simulink model "audio_setup"  (R2019b)
settings: Solver=FixedStepDiscrete  StartTime=0.0  StopTime=0.1  RelTol=1e-3
undefined symbols (not defined in the file): DiscIntNeverNeededParam
libraries: hdlsllib x15, simulink x11
settings Model: DataTypeOverride=Off  Creator=shahryar  LastModifiedBy=shahryar
settings SolverCC: AutoInsertRateTranBlk=on
settings DataIOCC: LimitDataPoints=on  SaveOutput=off  SaveTime=off
settings OptimizationCC: BlockReduction=off  ConditionallyExecuteInputs=off  DefaultParameterBehavior=Inlined  LifeSpan=inf
settings DebuggingCC: SignalRangeChecking=warning  AlgebraicLoopMsg=error  SingleTaskRateTransMsg=error  AllowSymbolicDim=off  StrictBusMsg=ErrorOnBusTreatedAsVector  SFUnexpectedBacktrackingDiag=warning  SFNoUnconditionalDefaultTransitionDiag=warning  SFExecutionAtInitializationDiag=none  ArithmeticOperatorsInVariantConditions=warning
settings HardwareCC: ProdBitPerPointer=32  ProdBitPerSizeT=32  ProdBitPerPtrDiffT=32  ProdLargestAtomicFloat=None  ProdIntDivRoundTo=Undefined  ProdEndianess=Unspecified  ProdWordSize=32  ProdHWDeviceType=ASIC/FPGA->ASIC/FPGA  TargetBitPerLong=64  TargetBitPerPointer=64  TargetBitPerSizeT=64  TargetBitPerPtrDiffT=64  TargetLongLongMode=on  TargetIntDivRoundTo=Zero  TargetEndianess=LittleEndian  TargetWordSize=64  TargetHWDeviceType=Custom Processor->MATLAB Host Computer  ProdEqTarget=off
settings SFSimCC: SimUseLocalCustomCode=off  CustomCodeUndefinedFunction=UseInterfaceOnly
settings RTWCC: RTWUseLocalCustomCode=off
settings CodeAppCC: StateflowObjectComments=on
settings GRTTargetCC: TargetLangStandard=C89/C90 (ANSI)  GeneratePreprocessorConditionals=Disable all
settings ConfigComp: CovScope=ReferencedModels  CovMetricSettings=dw  CovHtmlReporting=on  CovSaveCumulativeToWorkspaceVar=on  CovSaveSingleToWorkspaceVar=on  CovExternalEMLEnable=off  CovSFcnEnable=off

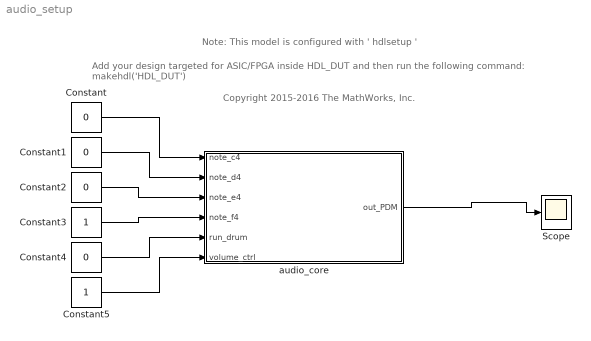
== system audio_setup ==
  note: Note: This model is configured with ' hdlsetup '
  note: Add your design targeted for ASIC/FPGA inside HDL_DUT and then run the following command:
      | makehdl('HDL_DUT')
  note: Copyright 2015-2016 The MathWorks, Inc.
  Constant{,1..2,4} (4 alike) : Constant  Value=0  OutDataTypeStr=boolean  SampleTime=1e-08
  Constant3 : Constant  OutDataTypeStr=boolean  SampleTime=1e-08
  Constant5 : Constant  OutDataTypeStr=fixdt(0,8,8)  SampleTime=1e-08
  Scope : Scope
  audio_core : Subsystem
  wires:
  Constant/1 -> audio_core/1(note_c4)
  Constant1/1 -> audio_core/2(note_d4)
  Constant2/1 -> audio_core/3(note_e4)
  Constant3/1 -> audio_core/4(note_f4)
  Constant4/1 -> audio_core/5(run_drum)
  Constant5/1 -> audio_core/6(volume_ctrl)
  audio_core/1(out_PDM) -> Scope/1

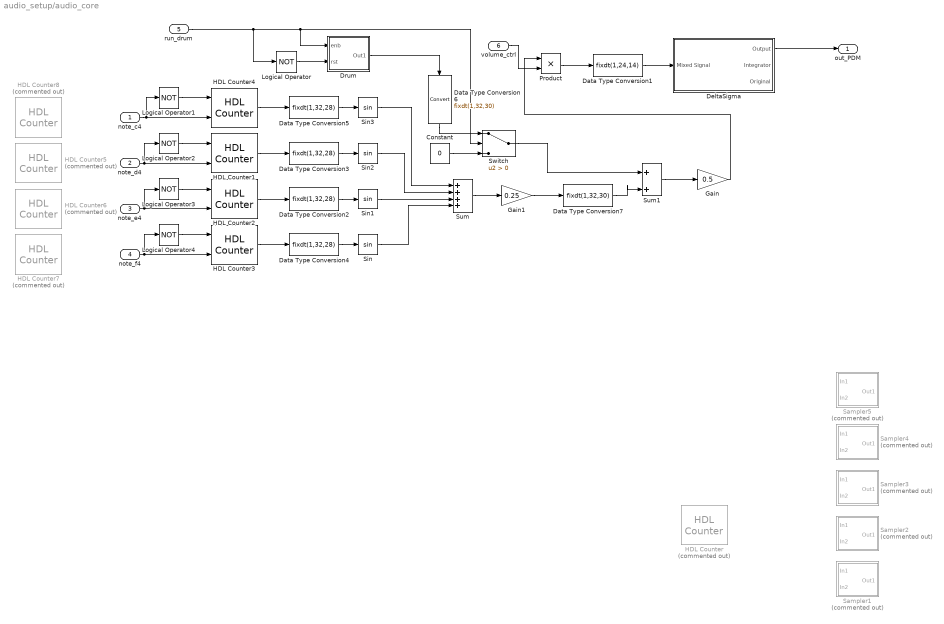
== system audio_setup/audio_core ==
  note_c4 : Inport
  note_d4 : Inport  Port=2
  note_e4 : Inport  Port=3
  note_f4 : Inport  Port=4
  run_drum : Inport  Port=5
  volume_ctrl : Inport  Port=6  OutDataTypeStr=fixdt(0,8,8)
  Constant : Constant  Value=0  OutDataTypeStr=fixdt(1,32,30)  SampleTime=1e-08
  Data Type Conversion1 : DataTypeConversion  OutDataTypeStr=fixdt(1,24,14)
  Data Type Conversion{2..5} (4 alike) : DataTypeConversion  OutDataTypeStr=fixdt(1,32,28)  ConvertRealWorld=Stored Integer (SI)
  Data Type Conversion6 : DataTypeConversion  OutDataTypeStr=fixdt(1,32,30)
  Data Type Conversion7 : DataTypeConversion  OutDataTypeStr=fixdt(1,32,30)
  DeltaSigma : Subsystem
  Drum : Subsystem
  Gain : Gain  Gain=0.5
  Gain1 : Gain  Gain=0.25
  HDL Counter : hdlsllib/Sources/HDL Counter  Commented=on  CountType=Count limited  CountInit=0  CountStep=1  CountMax=9  CountFromType=Initial value  CountFrom=0  CountResetPort=off  CountLoadPort=off  CountEnbPort=off  CountDirPort=off  CountDataType=Unsigned  CountWordLen=16  CountFracLen=0  CountSampTime=1e-08
      settings: SourceProductName=Simulink
  HDL Counter1 : hdlsllib/Sources/HDL Counter  CountType=Count limited  CountInit=3451652439+2218  CountStep=4953  CountMax=843314857-2218  CountFromType=Initial value  CountFrom=3451652439+2218  CountResetPort=on  CountLoadPort=off  CountEnbPort=on  CountDirPort=off  CountDataType=Unsigned  CountWordLen=32  CountFracLen=0  CountSampTime=1e-07
      settings: SourceProductName=Simulink
  HDL Counter2 : hdlsllib/Sources/HDL Counter  CountType=Count limited  CountInit=3451652439+1857  CountStep=5560  CountMax=843314857-1857  CountFromType=Initial value  CountFrom=3451652439+1857  CountResetPort=on  CountLoadPort=off  CountEnbPort=on  CountDirPort=off  CountDataType=Unsigned  CountWordLen=32  CountFracLen=0  CountSampTime=1e-07
      settings: SourceProductName=Simulink
  HDL Counter3 : hdlsllib/Sources/HDL Counter  CountType=Count limited  CountInit=3451652439+2327  CountStep=5890  CountMax=843314857-2327  CountFromType=Initial value  CountFrom=3451652439+2327  CountResetPort=on  CountLoadPort=off  CountEnbPort=on  CountDirPort=off  CountDataType=Unsigned  CountWordLen=32  CountFracLen=0  CountSampTime=1e-07
      settings: SourceProductName=Simulink
  HDL Counter4 : hdlsllib/Sources/HDL Counter  CountType=Count limited  CountInit=3451652439+1590  CountStep=4413  CountMax=843314857-1589  CountFromType=Initial value  CountFrom=3451652439+1590  CountResetPort=on  CountLoadPort=off  CountEnbPort=on  CountDirPort=off  CountDataType=Unsigned  CountWordLen=32  CountFracLen=0  CountSampTime=1e-07
      settings: SourceProductName=Simulink
  HDL Counter5 : hdlsllib/Sources/HDL Counter  Commented=on  CountType=Count limited  CountInit=3451652439+7171  CountStep=19812  CountMax=843314857-7171  CountFromType=Initial value  CountFrom=3451652439+7171  CountResetPort=on  CountLoadPort=off  CountEnbPort=on  CountDirPort=off  CountDataType=Unsigned  CountWordLen=32  CountFracLen=0  CountSampTime=1e-07
      settings: SourceProductName=Simulink
  HDL Counter6 : hdlsllib/Sources/HDL Counter  Commented=on  CountType=Count limited  CountInit=3451652439+5421  CountStep=22238  CountMax=843314857-5421  CountFromType=Initial value  CountFrom=3451652439+5421  CountResetPort=on  CountLoadPort=off  CountEnbPort=on  CountDirPort=off  CountDataType=Unsigned  CountWordLen=32  CountFracLen=0  CountSampTime=1e-07
      settings: SourceProductName=Simulink
  HDL Counter7 : hdlsllib/Sources/HDL Counter  Commented=on  CountType=Count limited  CountInit=3451652439+7765  CountStep=23561  CountMax=843314857-7764  CountFromType=Initial value  CountFrom=3451652439+7765  CountResetPort=on  CountLoadPort=off  CountEnbPort=on  CountDirPort=off  CountDataType=Unsigned  CountWordLen=32  CountFracLen=0  CountSampTime=1e-07
      settings: SourceProductName=Simulink
  HDL Counter8 : hdlsllib/Sources/HDL Counter  Commented=on  CountType=Count limited  CountInit=3451652439+3030  CountStep=17651  CountMax=843314857-3030  CountFromType=Initial value  CountFrom=3451652439+3030  CountResetPort=on  CountLoadPort=off  CountEnbPort=on  CountDirPort=off  CountDataType=Unsigned  CountWordLen=32  CountFracLen=0  CountSampTime=1e-07
      settings: SourceProductName=Simulink
  Logical Operator{,1..4} (5 alike) : Logic  Operator=NOT  IconShape=distinctive  AllPortsSameDT=off  OutDataTypeStr=boolean
  Product : Product
  Sampler1 : Subsystem  Commented=on
  Sampler2 : Subsystem  Commented=on
  Sampler3 : Subsystem  Commented=on
  Sampler4 : Subsystem  Commented=on
  Sampler5 : Subsystem  Commented=on
  Sin{,1..3} (4 alike) : Trigonometry  ApproximationMethod=CORDIC  NumberOfIterations=5  OutputSignalType=real
  Sum : Sum  Inputs=|+|+|+|+|
  Sum1 : Sum  Inputs=|+|+|
  Switch : Switch  Criteria=u2 > Threshold
  out_PDM : Outport  VectorParamsAs1DForOutWhenUnconnected=off
  wires:
  Data Type Conversion1/1 -> DeltaSigma/1(Mixed Signal)
  note_f4/1 -> Logical Operator4/1, HDL Counter3/2
  HDL Counter3/1 -> Data Type Conversion4/1
  Data Type Conversion4/1 -> Sin/1
  DeltaSigma/1(Output) -> out_PDM/1
  note_e4/1 -> Logical Operator3/1, HDL Counter2/2
  Data Type Conversion2/1 -> Sin1/1
  note_d4/1 -> Logical Operator2/1, HDL Counter1/2
  Data Type Conversion3/1 -> Sin2/1
  note_c4/1 -> Logical Operator1/1, HDL Counter4/2
  HDL Counter2/1 -> Data Type Conversion2/1
  HDL Counter1/1 -> Data Type Conversion3/1
  HDL Counter4/1 -> Data Type Conversion5/1
  Data Type Conversion5/1 -> Sin3/1
  run_drum/1 -> Logical Operator/1, Drum/1(enb), Switch/2
  Data Type Conversion6/1 -> Switch/1
  Constant/1 -> Switch/3
  Logical Operator1/1 -> HDL Counter4/1
  Logical Operator4/1 -> HDL Counter3/1
  Logical Operator3/1 -> HDL Counter2/1
  Logical Operator2/1 -> HDL Counter1/1
  Drum/1(Out1) -> Data Type Conversion6/1
  Logical Operator/1 -> Drum/2(rst)
  Gain/1 -> Product/1
  volume_ctrl/1 -> Product/2
  Product/1 -> Data Type Conversion1/1
  Sin3/1 -> Sum/1
  Sin2/1 -> Sum/2
  Sin1/1 -> Sum/3
  Sin/1 -> Sum/4
  Sum/1 -> Gain1/1
  Switch/1 -> Sum1/1
  Sum1/1 -> Gain/1
  Gain1/1 -> Data Type Conversion7/1
  Data Type Conversion7/1 -> Sum1/2

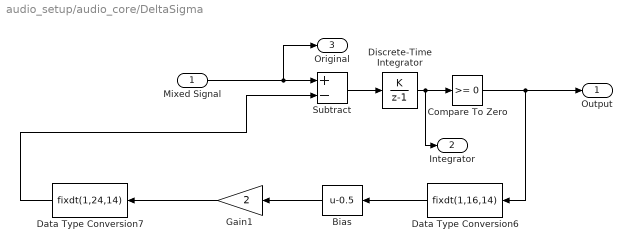
== system audio_setup/audio_core/DeltaSigma ==
  Mixed Signal : Inport
  Bias : Bias  Bias=-0.5
  Compare To Zero : simulink/Logic and Bit Operations/Compare To Zero  relop=>=  OutDataTypeStr=boolean
  Data Type Conversion6 : DataTypeConversion  OutDataTypeStr=fixdt(1,16,14)
  Data Type Conversion7 : DataTypeConversion  OutDataTypeStr=fixdt(1,24,14)
  Discrete-Time Integrator : DiscreteIntegrator  IntegratorMethod=Accumulation: Forward Euler  gainval=1  SampleTime=-1  OutDataTypeStr=fixdt(1,24,14)  UpperSaturationLimit=1  LowerSaturationLimit=-1  ICPrevOutput=DiscIntNeverNeededParam  ICPrevScaledInput=DiscIntNeverNeededParam
  Gain1 : Gain  Gain=2
  Subtract : Sum  Inputs=+-  AccumDataTypeStr=fixdt(1,16,12)  InputSameDT=on
  Output : Outport
  Integrator : Outport  Port=2  VectorParamsAs1DForOutWhenUnconnected=off
  Original : Outport  Port=3  VectorParamsAs1DForOutWhenUnconnected=off
  wires:
  Gain1/1 -> Data Type Conversion7/1
  Bias/1 -> Gain1/1
  Compare To Zero/1 -> Output/1, Data Type Conversion6/1
  Mixed Signal/1 -> Original/1, Subtract/1
  Data Type Conversion6/1 -> Bias/1
  Data Type Conversion7/1 -> Subtract/2
  Subtract/1 -> Discrete-Time Integrator/1
  Discrete-Time Integrator/1 -> Integrator/1, Compare To Zero/1

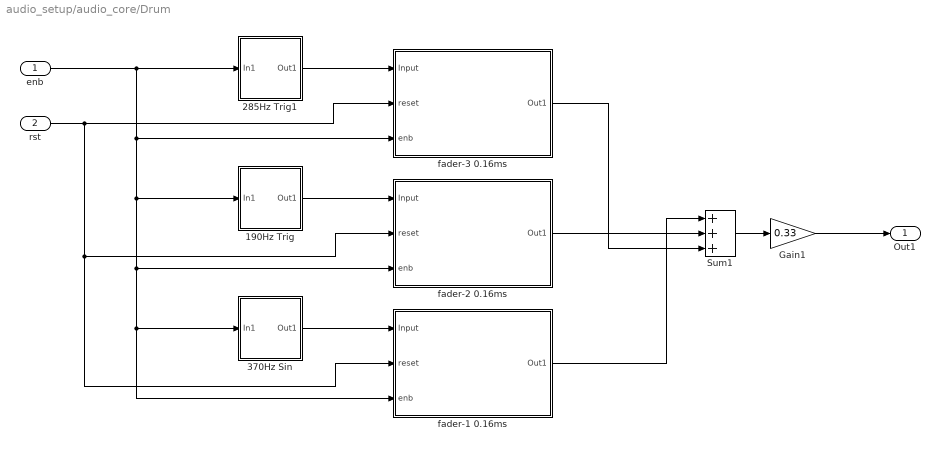
== system audio_setup/audio_core/Drum ==
  enb : Inport
  rst : Inport  Port=2
  190Hz Trig : Subsystem
  285Hz Trig1 : Subsystem
  370Hz Sin : Subsystem
  Gain1 : Gain  Gain=0.33
  Sum1 : Sum  Inputs=|+|+|+|
  fader-1 0.16ms : Subsystem
  fader-2 0.16ms : Subsystem
  fader-3 0.16ms : Subsystem
  Out1 : Outport
  wires:
  285Hz Trig1/1(Out1) -> fader-3 0.16ms/1(Input)
  Sum1/1 -> Gain1/1
  fader-2 0.16ms/1(Out1) -> Sum1/2
  370Hz Sin/1(Out1) -> fader-1 0.16ms/1(Input)
  190Hz Trig/1(Out1) -> fader-2 0.16ms/1(Input)
  fader-1 0.16ms/1(Out1) -> Sum1/1
  Gain1/1 -> Out1/1
  enb/1 -> 190Hz Trig/1(In1), fader-2 0.16ms/3(enb), fader-1 0.16ms/3(enb), 370Hz Sin/1(In1), fader-3 0.16ms/3(enb), 285Hz Trig1/1(In1)
  rst/1 -> fader-1 0.16ms/2(reset), fader-2 0.16ms/2(reset), fader-3 0.16ms/2(reset)
  fader-3 0.16ms/1(Out1) -> Sum1/3

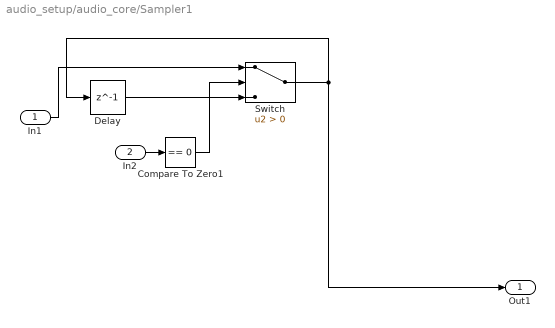
== system audio_setup/audio_core/Sampler1 ==
  In1 : Inport
  In2 : Inport  Port=2
  Compare To Zero1 : simulink/Logic and Bit Operations/Compare To Zero  relop===  OutDataTypeStr=boolean
  Delay : Delay  DelayLength=1  InitialCondition=1  UseCircularBuffer=on
  Switch : Switch  Criteria=u2 > Threshold
  Out1 : Outport
  wires:
  Delay/1 -> Switch/3
  In2/1 -> Compare To Zero1/1
  In1/1 -> Switch/1
  Switch/1 -> Out1/1, Delay/1
  Compare To Zero1/1 -> Switch/2

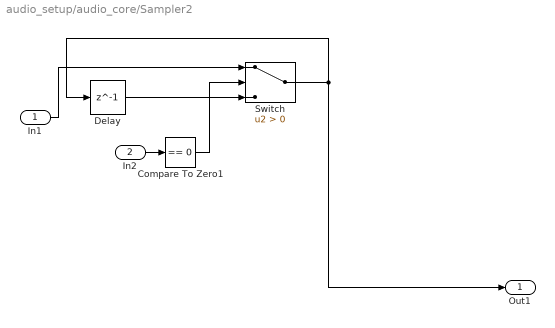
== system audio_setup/audio_core/Sampler2 ==
  In1 : Inport
  In2 : Inport  Port=2
  Compare To Zero1 : simulink/Logic and Bit Operations/Compare To Zero  relop===  OutDataTypeStr=boolean
  Delay : Delay  DelayLength=1  InitialCondition=1  UseCircularBuffer=on
  Switch : Switch  Criteria=u2 > Threshold
  Out1 : Outport
  wires:
  Delay/1 -> Switch/3
  In2/1 -> Compare To Zero1/1
  In1/1 -> Switch/1
  Switch/1 -> Out1/1, Delay/1
  Compare To Zero1/1 -> Switch/2

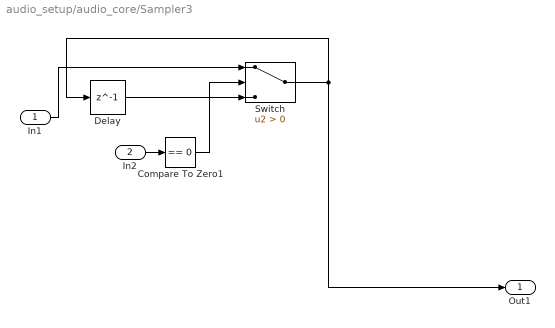
== system audio_setup/audio_core/Sampler3 ==
  In1 : Inport
  In2 : Inport  Port=2
  Compare To Zero1 : simulink/Logic and Bit Operations/Compare To Zero  relop===  OutDataTypeStr=boolean
  Delay : Delay  DelayLength=1  InitialCondition=1  UseCircularBuffer=on
  Switch : Switch  Criteria=u2 > Threshold
  Out1 : Outport
  wires:
  Delay/1 -> Switch/3
  In2/1 -> Compare To Zero1/1
  In1/1 -> Switch/1
  Switch/1 -> Out1/1, Delay/1
  Compare To Zero1/1 -> Switch/2

== system audio_setup/audio_core/Sampler4 ==
  In1 : Inport
  In2 : Inport  Port=2
  Compare To Zero1 : simulink/Logic and Bit Operations/Compare To Zero  relop===  OutDataTypeStr=boolean
  Delay : Delay  DelayLength=1  InitialCondition=1  UseCircularBuffer=on
  Switch : Switch  Criteria=u2 > Threshold
  Out1 : Outport
  wires:
  Delay/1 -> Switch/3
  In2/1 -> Compare To Zero1/1
  In1/1 -> Switch/1
  Switch/1 -> Out1/1, Delay/1
  Compare To Zero1/1 -> Switch/2

== system audio_setup/audio_core/Sampler5 ==
  In1 : Inport
  In2 : Inport  Port=2
  Compare To Zero1 : simulink/Logic and Bit Operations/Compare To Zero  relop===  OutDataTypeStr=boolean
  Delay : Delay  DelayLength=1  InitialCondition=1  UseCircularBuffer=on
  Switch : Switch  Criteria=u2 > Threshold
  Out1 : Outport
  wires:
  Delay/1 -> Switch/3
  In2/1 -> Compare To Zero1/1
  In1/1 -> Switch/1
  Switch/1 -> Out1/1, Delay/1
  Compare To Zero1/1 -> Switch/2

== system audio_setup/audio_core/Drum/190Hz Trig ==
  In1 : Inport
  Data Type Conversion6 : DataTypeConversion  OutDataTypeStr=fixdt(1,22,18)  ConvertRealWorld=Stored Integer (SI)
  Data Type Conversion7 : DataTypeConversion  OutDataTypeStr=fixdt(1,20,16)
  HDL Counter6 : hdlsllib/Sources/HDL Counter  CountType=Count limited  CountInit=0  CountStep=1  CountMax=262144  CountFromType=Initial value  CountFrom=0  CountResetPort=off  CountLoadPort=off  CountEnbPort=on  CountDirPort=off  CountDataType=Unsigned  CountWordLen=22  CountFracLen=0  CountSampTime=1
      settings: SourceProductName=Simulink
  Trig1 : Subsystem
  Out1 : Outport
  wires:
  In1/1 -> HDL Counter6/1
  HDL Counter6/1 -> Trig1/1(In1), Data Type Conversion6/1
  Data Type Conversion6/1 -> Trig1/2(In2)
  Data Type Conversion7/1 -> Out1/1
  Trig1/1(Out1) -> Data Type Conversion7/1

== system audio_setup/audio_core/Drum/285Hz Trig1 ==
  In1 : Inport
  Data Type Conversion6 : DataTypeConversion  OutDataTypeStr=fixdt(1,23,19)  ConvertRealWorld=Stored Integer (SI)
  Data Type Conversion7 : DataTypeConversion  OutDataTypeStr=fixdt(1,20,16)
  HDL Counter6 : hdlsllib/Sources/HDL Counter  CountType=Count limited  CountInit=0  CountStep=3  CountMax=524286  CountFromType=Initial value  CountFrom=0  CountResetPort=off  CountLoadPort=off  CountEnbPort=on  CountDirPort=off  CountDataType=Unsigned  CountWordLen=23  CountFracLen=0  CountSampTime=1
      settings: SourceProductName=Simulink
  Trig1 : Subsystem
  Out1 : Outport
  wires:
  In1/1 -> HDL Counter6/1
  HDL Counter6/1 -> Trig1/1(In1), Data Type Conversion6/1
  Data Type Conversion6/1 -> Trig1/2(In2)
  Data Type Conversion7/1 -> Out1/1
  Trig1/1(Out1) -> Data Type Conversion7/1

== system audio_setup/audio_core/Drum/370Hz Sin ==
  In1 : Inport
  Data Type Conversion6 : DataTypeConversion  OutDataTypeStr=fixdt(1,21,17)  ConvertRealWorld=Stored Integer (SI)
  Data Type Conversion7 : DataTypeConversion  OutDataTypeStr=fixdt(1,20,18)
  HDL Counter5 : hdlsllib/Sources/HDL Counter  CountType=Count limited  CountInit=1685377  CountStep=3  CountMax=411773  CountFromType=Initial value  CountFrom=1685377  CountResetPort=off  CountLoadPort=off  CountEnbPort=on  CountDirPort=off  CountDataType=Unsigned  CountWordLen=21  CountFracLen=0  CountSampTime=1e-07
      settings: SourceProductName=Simulink
  Sin4 : Trigonometry  ApproximationMethod=CORDIC  NumberOfIterations=5  OutputSignalType=real
  Out1 : Outport
  wires:
  HDL Counter5/1 -> Data Type Conversion6/1
  Sin4/1 -> Data Type Conversion7/1
  Data Type Conversion6/1 -> Sin4/1
  In1/1 -> HDL Counter5/1
  Data Type Conversion7/1 -> Out1/1

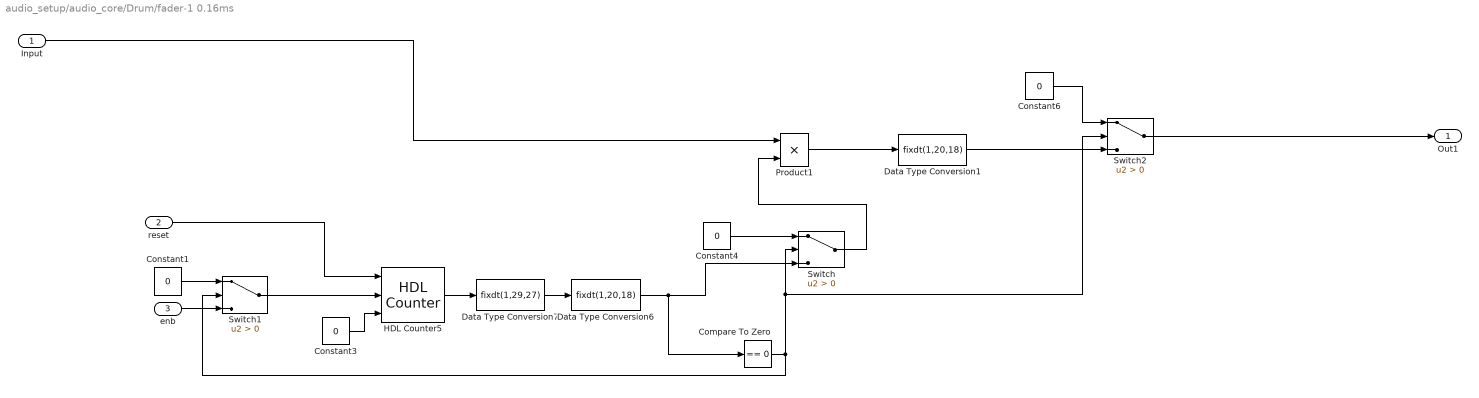
== system audio_setup/audio_core/Drum/fader-1 0.16ms ==
  Input : Inport
  reset : Inport  Port=2
  enb : Inport  Port=3
  Compare To Zero : simulink/Logic and Bit Operations/Compare To Zero  relop===  OutDataTypeStr=boolean
  Constant1 : Constant  Value=0  OutDataTypeStr=boolean  SampleTime=1e-08
  Constant3 : Constant  Value=0  OutDataTypeStr=boolean  SampleTime=1e-08
  Constant4 : Constant  Value=0  OutDataTypeStr=fixdt(1,20,18)  SampleTime=1e-08
  Constant6 : Constant  Value=0  OutDataTypeStr=fixdt(1,20,18)  SampleTime=1e-08
  Data Type Conversion1 : DataTypeConversion  OutDataTypeStr=fixdt(1,20,18)
  Data Type Conversion6 : DataTypeConversion  OutDataTypeStr=fixdt(1,20,18)
  Data Type Conversion7 : DataTypeConversion  OutDataTypeStr=fixdt(1,29,27)  ConvertRealWorld=Stored Integer (SI)
  HDL Counter5 : hdlsllib/Sources/HDL Counter  CountType=Count limited  CountInit=134217728  CountStep=8  CountMax=0  CountFromType=Specify  CountFrom=134217728  CountResetPort=on  CountLoadPort=off  CountEnbPort=on  CountDirPort=on  CountDataType=Unsigned  CountWordLen=29  CountFracLen=0  CountSampTime=1e-07
      settings: SourceProductName=Simulink
  Product1 : Product
  Switch : Switch  Criteria=u2 > Threshold
  Switch1 : Switch  Criteria=u2 > Threshold
  Switch2 : Switch  Criteria=u2 > Threshold
  Out1 : Outport
  wires:
  Switch/1 -> Product1/2
  Data Type Conversion6/1 -> Compare To Zero/1, Switch/3
  Compare To Zero/1 -> Switch2/2, Switch/2, Switch1/2
  Constant6/1 -> Switch2/1
  Data Type Conversion7/1 -> Data Type Conversion6/1
  Constant4/1 -> Switch/1
  Switch1/1 -> HDL Counter5/2
  Switch2/1 -> Out1/1
  Input/1 -> Product1/1
  reset/1 -> HDL Counter5/1
  HDL Counter5/1 -> Data Type Conversion7/1
  Constant3/1 -> HDL Counter5/3
  Constant1/1 -> Switch1/1
  enb/1 -> Switch1/3
  Product1/1 -> Data Type Conversion1/1
  Data Type Conversion1/1 -> Switch2/3

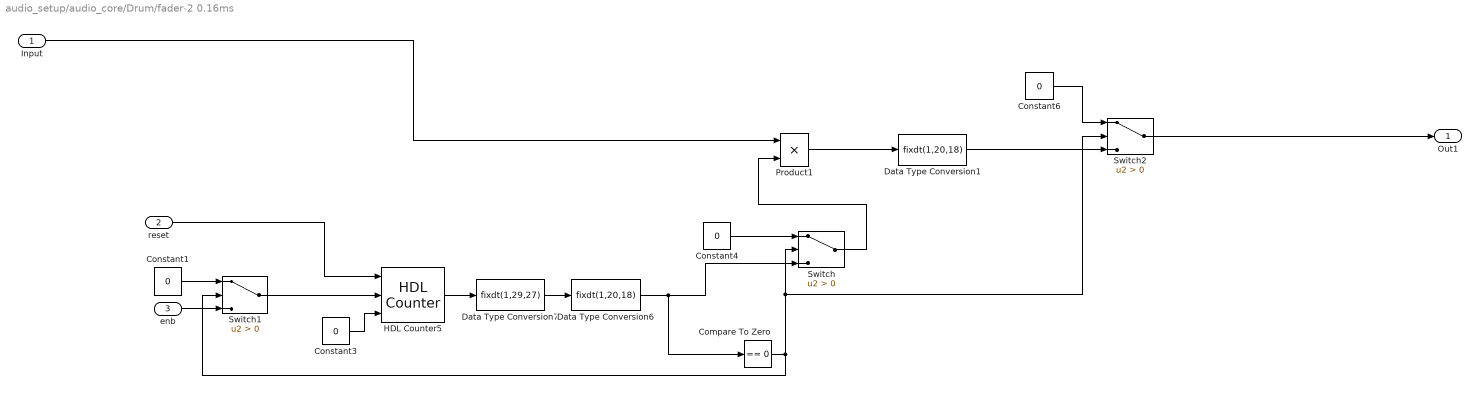
== system audio_setup/audio_core/Drum/fader-2 0.16ms ==
  Input : Inport
  reset : Inport  Port=2
  enb : Inport  Port=3
  Compare To Zero : simulink/Logic and Bit Operations/Compare To Zero  relop===  OutDataTypeStr=boolean
  Constant1 : Constant  Value=0  OutDataTypeStr=boolean  SampleTime=1e-08
  Constant3 : Constant  Value=0  OutDataTypeStr=boolean  SampleTime=1e-08
  Constant4 : Constant  Value=0  OutDataTypeStr=fixdt(1,20,18)  SampleTime=1e-08
  Constant6 : Constant  Value=0  OutDataTypeStr=fixdt(1,20,18)  SampleTime=1e-08
  Data Type Conversion1 : DataTypeConversion  OutDataTypeStr=fixdt(1,20,18)
  Data Type Conversion6 : DataTypeConversion  OutDataTypeStr=fixdt(1,20,18)
  Data Type Conversion7 : DataTypeConversion  OutDataTypeStr=fixdt(1,29,27)  ConvertRealWorld=Stored Integer (SI)
  HDL Counter5 : hdlsllib/Sources/HDL Counter  CountType=Count limited  CountInit=134217728  CountStep=8  CountMax=0  CountFromType=Specify  CountFrom=134217728  CountResetPort=on  CountLoadPort=off  CountEnbPort=on  CountDirPort=on  CountDataType=Unsigned  CountWordLen=29  CountFracLen=0  CountSampTime=1e-07
      settings: SourceProductName=Simulink
  Product1 : Product
  Switch : Switch  Criteria=u2 > Threshold
  Switch1 : Switch  Criteria=u2 > Threshold
  Switch2 : Switch  Criteria=u2 > Threshold
  Out1 : Outport
  wires:
  Switch/1 -> Product1/2
  Data Type Conversion6/1 -> Compare To Zero/1, Switch/3
  Compare To Zero/1 -> Switch2/2, Switch/2, Switch1/2
  Constant6/1 -> Switch2/1
  Data Type Conversion7/1 -> Data Type Conversion6/1
  Constant4/1 -> Switch/1
  Switch1/1 -> HDL Counter5/2
  Switch2/1 -> Out1/1
  Input/1 -> Product1/1
  reset/1 -> HDL Counter5/1
  HDL Counter5/1 -> Data Type Conversion7/1
  Constant3/1 -> HDL Counter5/3
  Constant1/1 -> Switch1/1
  enb/1 -> Switch1/3
  Product1/1 -> Data Type Conversion1/1
  Data Type Conversion1/1 -> Switch2/3

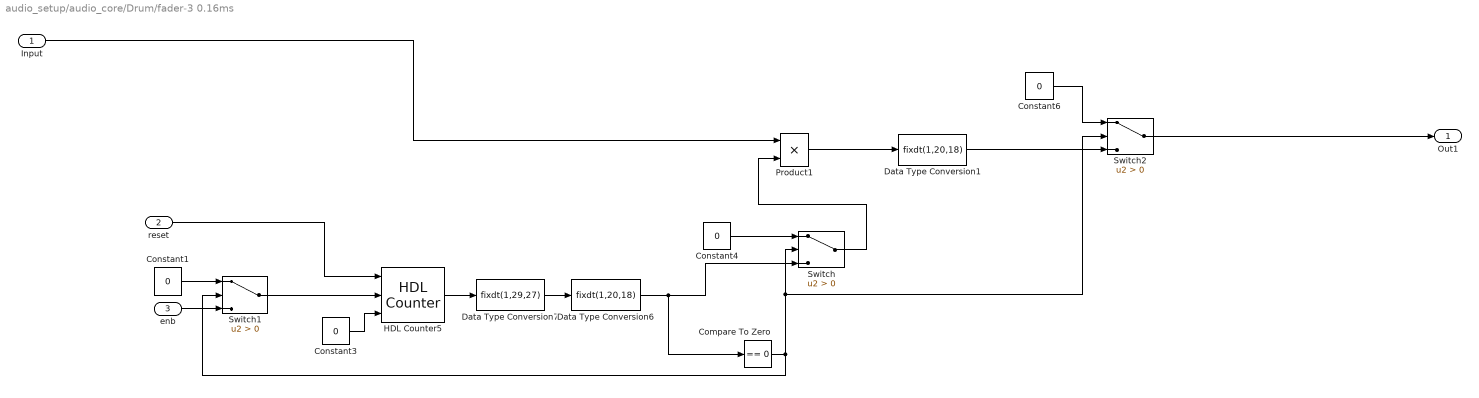
== system audio_setup/audio_core/Drum/fader-3 0.16ms ==
  Input : Inport
  reset : Inport  Port=2
  enb : Inport  Port=3
  Compare To Zero : simulink/Logic and Bit Operations/Compare To Zero  relop===  OutDataTypeStr=boolean
  Constant1 : Constant  Value=0  OutDataTypeStr=boolean  SampleTime=1e-08
  Constant3 : Constant  Value=0  OutDataTypeStr=boolean  SampleTime=1e-08
  Constant4 : Constant  Value=0  OutDataTypeStr=fixdt(1,20,18)  SampleTime=1e-08
  Constant6 : Constant  Value=0  OutDataTypeStr=fixdt(1,20,18)  SampleTime=1e-08
  Data Type Conversion1 : DataTypeConversion  OutDataTypeStr=fixdt(1,20,18)
  Data Type Conversion6 : DataTypeConversion  OutDataTypeStr=fixdt(1,20,18)
  Data Type Conversion7 : DataTypeConversion  OutDataTypeStr=fixdt(1,29,27)  ConvertRealWorld=Stored Integer (SI)
  HDL Counter5 : hdlsllib/Sources/HDL Counter  CountType=Count limited  CountInit=134217728  CountStep=8  CountMax=0  CountFromType=Specify  CountFrom=134217728  CountResetPort=on  CountLoadPort=off  CountEnbPort=on  CountDirPort=on  CountDataType=Unsigned  CountWordLen=29  CountFracLen=0  CountSampTime=1e-07
      settings: SourceProductName=Simulink
  Product1 : Product
  Switch : Switch  Criteria=u2 > Threshold
  Switch1 : Switch  Criteria=u2 > Threshold
  Switch2 : Switch  Criteria=u2 > Threshold
  Out1 : Outport
  wires:
  Switch/1 -> Product1/2
  Data Type Conversion6/1 -> Compare To Zero/1, Switch/3
  Compare To Zero/1 -> Switch2/2, Switch/2, Switch1/2
  Constant6/1 -> Switch2/1
  Data Type Conversion7/1 -> Data Type Conversion6/1
  Constant4/1 -> Switch/1
  Switch1/1 -> HDL Counter5/2
  Switch2/1 -> Out1/1
  Input/1 -> Product1/1
  reset/1 -> HDL Counter5/1
  HDL Counter5/1 -> Data Type Conversion7/1
  Constant3/1 -> HDL Counter5/3
  Constant1/1 -> Switch1/1
  enb/1 -> Switch1/3
  Product1/1 -> Data Type Conversion1/1
  Data Type Conversion1/1 -> Switch2/3

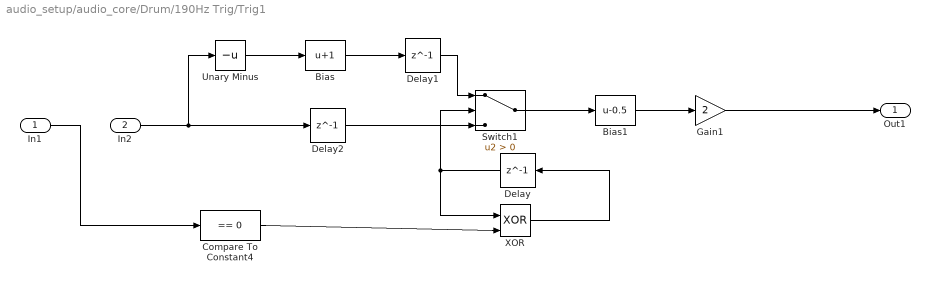
== system audio_setup/audio_core/Drum/190Hz Trig/Trig1 ==
  In1 : Inport
  In2 : Inport  Port=2
  Bias : Bias  Bias=1
  Bias1 : Bias  Bias=-0.5
  Compare To Constant4 : simulink/Logic and Bit Operations/Compare To Constant  relop===  const=0  OutDataTypeStr=boolean
  Delay : Delay  DelayLength=1  InitialCondition=0
  Delay1 : Delay  DelayLength=1  InitialCondition=0
  Delay2 : Delay  DelayLength=1  InitialCondition=0
  Gain1 : Gain  Gain=2
  Switch1 : Switch  Criteria=u2 > Threshold
  Unary Minus : UnaryMinus
  XOR : Logic  Operator=XOR  IconShape=distinctive  AllPortsSameDT=off  OutDataTypeStr=boolean
  Out1 : Outport
  wires:
  Unary Minus/1 -> Bias/1
  XOR/1 -> Delay/1
  Compare To Constant4/1 -> XOR/2
  Switch1/1 -> Bias1/1
  Delay2/1 -> Switch1/3
  Gain1/1 -> Out1/1
  Delay1/1 -> Switch1/1
  Delay/1 -> XOR/1, Switch1/2
  Bias/1 -> Delay1/1
  Bias1/1 -> Gain1/1
  In1/1 -> Compare To Constant4/1
  In2/1 -> Delay2/1, Unary Minus/1

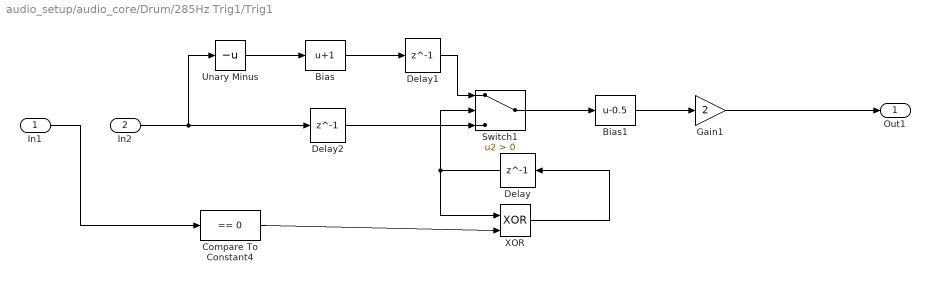
== system audio_setup/audio_core/Drum/285Hz Trig1/Trig1 ==
  In1 : Inport
  In2 : Inport  Port=2
  Bias : Bias  Bias=1
  Bias1 : Bias  Bias=-0.5
  Compare To Constant4 : simulink/Logic and Bit Operations/Compare To Constant  relop===  const=0  OutDataTypeStr=boolean
  Delay : Delay  DelayLength=1  InitialCondition=0
  Delay1 : Delay  DelayLength=1  InitialCondition=0
  Delay2 : Delay  DelayLength=1  InitialCondition=0
  Gain1 : Gain  Gain=2
  Switch1 : Switch  Criteria=u2 > Threshold
  Unary Minus : UnaryMinus
  XOR : Logic  Operator=XOR  IconShape=distinctive  AllPortsSameDT=off  OutDataTypeStr=boolean
  Out1 : Outport
  wires:
  Unary Minus/1 -> Bias/1
  XOR/1 -> Delay/1
  Compare To Constant4/1 -> XOR/2
  Switch1/1 -> Bias1/1
  Delay2/1 -> Switch1/3
  Gain1/1 -> Out1/1
  Delay1/1 -> Switch1/1
  Delay/1 -> XOR/1, Switch1/2
  Bias/1 -> Delay1/1
  Bias1/1 -> Gain1/1
  In1/1 -> Compare To Constant4/1
  In2/1 -> Delay2/1, Unary Minus/1
